simulink model "XGGDZhPIDzls"  (Simulink 5.0)
settings: Solver=ode4  StartTime=0.0  StopTime=8000  FixedStep=20  RelTol=1e-3
settings Model: LastModifiedBy=ThinkPad

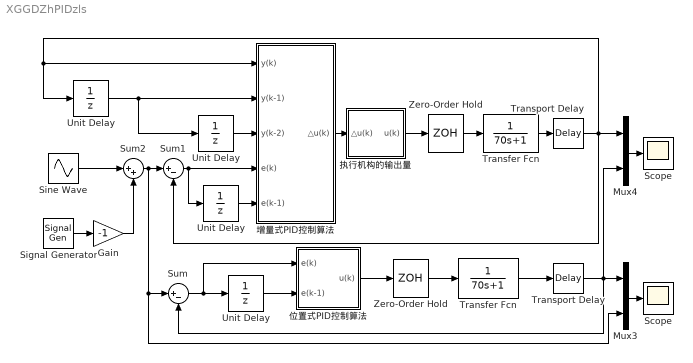
== system XGGDZhPIDzls ==
  " Unit Delay" : UnitDelay  SampleTime=20
  " Unit Delay " : UnitDelay  SampleTime=20
  Gain : Gain  Gain=-1  SaturateOnIntegerOverflow=on
  Mux3 : Mux  Inputs=2
  Mux4 : Mux  Inputs=2
  Scope : Scope
      settings: YMin=-1.3  YMax=1.3  MaxDataPoints=500000
  "Scope " : Scope
      settings: YMin=-1.3  YMax=1.3  SaveName=PID  DataFormat=Array  MaxDataPoints=500000
  "Signal Generator " : SignalGenerator  WaveForm=square  Frequency=0.0005*pi  Units=rad/sec
  "Sine Wave " : Sin  Amplitude=0.05  Frequency=0.03*pi  SampleTime=0
  Sum : Sum  Inputs=|+-  SaturateOnIntegerOverflow=on
  Sum1 : Sum  Inputs=|+-  SaturateOnIntegerOverflow=on
  Sum2 : Sum  Inputs=|++  SaturateOnIntegerOverflow=on
  Transfer Fcn : TransferFcn  Denominator=[70 1]
  "Transfer Fcn " : TransferFcn  Denominator=[70 1]
  Transport Delay : TransportDelay  DelayTime=80
  "Transport Delay " : TransportDelay  DelayTime=80
  Unit Delay : UnitDelay  SampleTime=20
  "Unit Delay " : UnitDelay  SampleTime=20
  Zero-Order Hold : ZeroOrderHold  SampleTime=20
  "Zero-Order Hold " : ZeroOrderHold  SampleTime=20
  "位置式PID控制算法 " : Subsystem
  增量式PID控制算法 : Subsystem
  执行机构的输出量 : Subsystem
  wires:
  "Sine Wave "/1 -> Sum2/1
  "Signal Generator "/1 -> Gain/1
  Gain/1 -> Sum2/2
  Sum2/1 -> Sum1/1, Sum/1, Mux3/2
  Sum/1 -> Unit Delay/1, "位置式PID控制算法 "/1(e(k))
  "位置式PID控制算法 "/1(u(k)) -> "Zero-Order Hold "/1
  Mux3/1 -> "Scope "/1
  "Transfer Fcn "/1 -> "Transport Delay "/1
  "Zero-Order Hold "/1 -> "Transfer Fcn "/1
  "Transport Delay "/1 -> Sum/2, Mux3/1, Mux4/2
  Unit Delay/1 -> "位置式PID控制算法 "/2(e(k-1))
  Transfer Fcn/1 -> Transport Delay/1
  Zero-Order Hold/1 -> Transfer Fcn/1
  Mux4/1 -> Scope/1
  Transport Delay/1 -> Sum1/2, Mux4/1, " Unit Delay "/1, 增量式PID控制算法/1(y(k))
  增量式PID控制算法/1("△u(k) ") -> 执行机构的输出量/1("△u(k) ")
  执行机构的输出量/1(u(k)) -> Zero-Order Hold/1
  Sum1/1 -> 增量式PID控制算法/4(e(k)), "Unit Delay "/1
  "Unit Delay "/1 -> 增量式PID控制算法/5(e(k-1))
  " Unit Delay "/1 -> 增量式PID控制算法/2(y(k-1)), " Unit Delay"/1
  " Unit Delay"/1 -> 增量式PID控制算法/3(y(k-2))

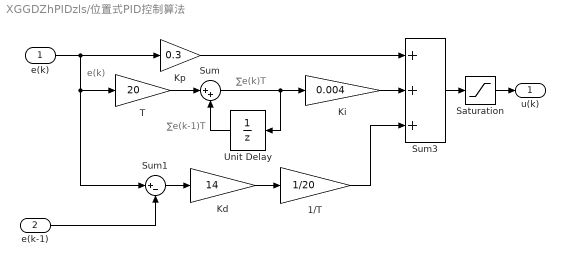
== system XGGDZhPIDzls/位置式PID控制算法  ==
  note: e(k)
  note: ∑e(k)T
  note: ∑e(k-1)T
  e(k) : Inport
  e(k-1) : Inport  Port=2
  1/T : Gain  Gain=1/20  SaturateOnIntegerOverflow=on
  Kd : Gain  Gain=14  SaturateOnIntegerOverflow=on
  Ki : Gain  Gain=0.004  SaturateOnIntegerOverflow=on
  Kp : Gain  Gain=0.3  SaturateOnIntegerOverflow=on
  Saturation : Saturate  UpperLimit=10  LowerLimit=-10
  Sum : Sum  Inputs=|++  SaturateOnIntegerOverflow=on
  Sum1 : Sum  Inputs=|+-  SaturateOnIntegerOverflow=on
  Sum3 : Sum  Inputs=+++  SaturateOnIntegerOverflow=on
  T : Gain  Gain=20  SaturateOnIntegerOverflow=on
  Unit Delay : UnitDelay  Orientation=left  SampleTime=20
  u(k) : Outport
  wires:
  Sum1/1 -> Kd/1
  e(k)/1 -> Kp/1, Sum1/1, T/1
  Kp/1 -> Sum3/1
  Ki/1 -> Sum3/2
  Sum3/1 -> Saturation/1
  Kd/1 -> 1/T/1
  1/T/1 -> Sum3/3
  Sum/1 -> Unit Delay/1, Ki/1
  Unit Delay/1 -> Sum/2
  e(k-1)/1 -> Sum1/2
  T/1 -> Sum/1
  Saturation/1 -> u(k)/1

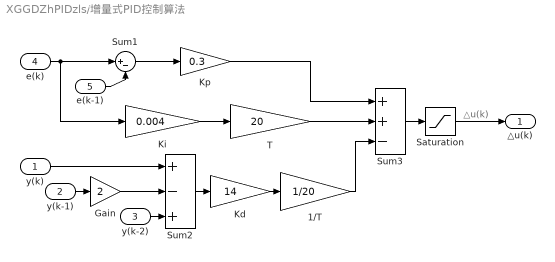
== system XGGDZhPIDzls/增量式PID控制算法 ==
  note: △u(k)
  y(k) : Inport
  y(k-1) : Inport  Port=2
  y(k-2) : Inport  Port=3
  e(k) : Inport  Port=4
  e(k-1) : Inport  Port=5
  1/T : Gain  Gain=1/20  SaturateOnIntegerOverflow=on
  Gain : Gain  Gain=2  SaturateOnIntegerOverflow=on
  Kd : Gain  Gain=14  SaturateOnIntegerOverflow=on
  Ki : Gain  Gain=0.004  SaturateOnIntegerOverflow=on
  Kp : Gain  Gain=0.3  SaturateOnIntegerOverflow=on
  Saturation : Saturate  UpperLimit=10  LowerLimit=-10
  Sum1 : Sum  Inputs=|+-  SaturateOnIntegerOverflow=on
  Sum2 : Sum  Inputs=+-+  SaturateOnIntegerOverflow=on
  Sum3 : Sum  Inputs=++-  SaturateOnIntegerOverflow=on
  T : Gain  Gain=20  SaturateOnIntegerOverflow=on
  "△u(k) " : Outport
  wires:
  Sum1/1 -> Kp/1
  Gain/1 -> Sum2/2
  Sum2/1 -> Kd/1
  e(k-1)/1 -> Sum1/2
  y(k-2)/1 -> Sum2/3
  e(k)/1 -> Sum1/1, Ki/1
  Kp/1 -> Sum3/1
  Ki/1 -> T/1
  Sum3/1 -> Saturation/1
  Kd/1 -> 1/T/1
  T/1 -> Sum3/2
  1/T/1 -> Sum3/3
  y(k)/1 -> Sum2/1
  y(k-1)/1 -> Gain/1
  Saturation/1 -> "△u(k) "/1

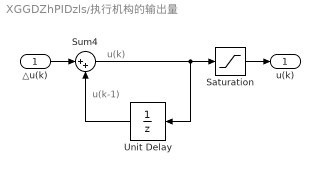
== system XGGDZhPIDzls/执行机构的输出量 ==
  note: u(k-1)
  note: u(k)
  "△u(k) " : Inport
  Saturation : Saturate  UpperLimit=10  LowerLimit=-10
  Sum4 : Sum  Inputs=|++  SaturateOnIntegerOverflow=on
  Unit Delay : UnitDelay  Orientation=left  SampleTime=20
  u(k) : Outport
  wires:
  Sum4/1 -> Saturation/1, Unit Delay/1
  Unit Delay/1 -> Sum4/2
  "△u(k) "/1 -> Sum4/1
  Saturation/1 -> u(k)/1
